simulink library "mpc_lib"  (Simulink 6.4)
libraries: simulink x1
settings Model: LastModifiedBy=Developer

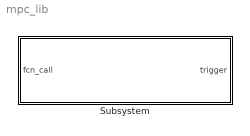
== system mpc_lib ==
  Subsystem : Subsystem  TreatAsAtomicUnit=on  mask{trig_len=0.02}
      mask prompts: trig_len "Otuput trigger length"
      mask Display:
      | disp('fcn_call_to_rising_edge');
      | port_label('output', 1, 'trigger');
      | port_label('input', 1, 'fcn_call');

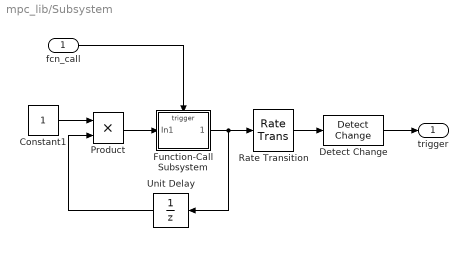
== system mpc_lib/Subsystem ==
  fcn_call : Inport
  Constant1 : Constant  Value=1  OutDataType=sfix(16)  ConRadixGroup=Use specified scaling  OutScaling=2^0  SampleTime=inf  FramePeriod=inf
  Detect Change : simulink/Logic and Bit Operations/Detect Change  SystemSampleTime=-1  vinit=1
  Function-Call Subsystem : Subsystem  TreatAsAtomicUnit=on
  Product : Product  RndMeth=Zero
  Rate Transition : RateTransition  X0=1  OutPortSampleTime=trig_len
  Unit Delay : UnitDelay  Orientation=left  X0=1  SampleTime=-1
  trigger : Outport
  wires:
  fcn_call/1 -> Function-Call Subsystem/Trigger
  Function-Call Subsystem/1(trigger1) -> Rate Transition/1, Unit Delay/1
  Constant1/1 -> Product/1
  Unit Delay/1 -> Product/2
  Product/1 -> Function-Call Subsystem/1(In1)
  Rate Transition/1 -> Detect Change/1
  Detect Change/1 -> trigger/1

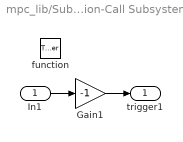
== system mpc_lib/Subsystem/Function-Call Subsystem ==
  In1 : Inport
  function : TriggerPort  TriggerType=function-call  SampleTime=-1
  Gain1 : Gain  Gain=-1
  trigger1 : Outport
  wires:
  In1/1 -> Gain1/1
  Gain1/1 -> trigger1/1
